simulink model "Rider_Controls_OutHardware"  (R2014b)
settings: configuration reference "Embedded_Configuration" (kept outside this file)
PostLoadFcn:
  | load('Embedded_Config.mat')
model workspace: external: MAT-File Embedded_Config.mat (data not in the file)
libraries: canmsglib x2, c280xlib x2
settings Model: Creator=The MathWorks Inc.  LastModifiedBy=Sean

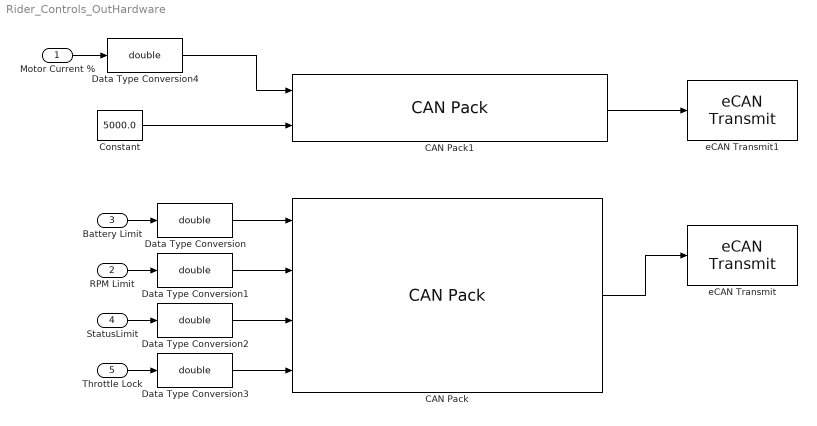
== system Rider_Controls_OutHardware ==
  Motor Current % : Inport  OutDataTypeStr=single
  RPM Limit : Inport  Port=2  OutDataTypeStr=uint16
  Battery Limit : Inport  Port=3  OutDataTypeStr=uint16
  StatusLimit : Inport  Port=4  OutDataTypeStr=uint16
  Throttle Lock : Inport  Port=5  OutDataTypeStr=uint16
  CAN Pack : canmsglib/CAN Pack  CANdbFile=C:\Users\Sean\Desktop\Buckeye Current\Databases\RW3.dbc  MsgList=DriveControlsLimits  MsgName=DriveControlsLimits  MsgIDType=Standard (11-bit identifier)  MsgIdentifier=483  MsgLength=8  SignalInfo=BatteryLimit$1$1$1$2$1$0$1$0$0$1$#RPMLimit$2$1$1$2$1$0$1$0$0$1$#StatusLimit$3$1$1$2$1$0$1$0$-Inf$Inf$#ThrottleLock$0$1$1$2$1$0$1$0$-Inf$Inf$#  NSignals=4  StartBits=str2num('[int32(1);int32(2);int32(3);int32(0)]')  SignalSizes=str2num('[int32(1);int32(1);int32(1);int32(1)]')  ByteOrders=str2num('[int32(1);int32(1);int32(1);int32(1)]')  DataTypes=str2num('[int32(2);int32(2);int32(2);int32(2)]')  MultiplexTypes=str2num('[int32(1);int32(1);int32(1);int32(1)]')  MultiplexValues=str2num('[double(0);double(0);double(0);double(0)]')  Factors=str2num('[double(1);double(1);double(1);double(1)]')  Offsets=str2num('[double(0);double(0);double(0);double(0)]')  Minimums=str2num('[double(0);double(0);double(-Inf);double(-Inf)]')  Maximums=str2num('[double(1);double(1);double(Inf);double(Inf)]')  Remote=off
      settings: DataFormat=CANdb specified signals
  CAN Pack1 : canmsglib/CAN Pack  CANdbFile=C:\Users\Sean\Desktop\Buckeye Current\Databases\RW3.dbc  MsgList=MotorDriveCommand  MsgName=MotorDriveCommand  MsgIDType=Standard (11-bit identifier)  MsgIdentifier=480  MsgLength=8  SignalInfo=MotorCurrentSetpoint$32$32$1$3$1$0$1$0$0$1$#MotorRPMSetpoint$0$32$1$3$1$0$1$0$0$4000$#  NSignals=2  StartBits=str2num('[int32(32);int32(0)]')  SignalSizes=str2num('[int32(32);int32(32)]')  ByteOrders=str2num('[int32(1);int32(1)]')  DataTypes=str2num('[int32(3);int32(3)]')  MultiplexTypes=str2num('[int32(1);int32(1)]')  MultiplexValues=str2num('[double(0);double(0)]')  Factors=str2num('[double(1);double(1)]')  Offsets=str2num('[double(0);double(0)]')  Minimums=str2num('[double(0);double(0)]')  Maximums=str2num('[double(1);double(4000)]')  Remote=off
      settings: DataFormat=CANdb specified signals
  Constant : Constant  Value=5000.0  OutDataTypeStr=Inherit: Inherit via back propagation  SampleTime=0.01
  Data Type Conversion{,1..4} (5 alike) : DataTypeConversion  OutDataTypeStr=double
  eCAN Transmit : c280xlib/eCAN Transmit  chipFamily=C280x  useModule=eCAN_A  mailboxNo=31  messageID=483  messageType=Standard (11-bit identifier)  enableBlockingMode=off  postInterrupt=off  interruptLine=0
  eCAN Transmit1 : c280xlib/eCAN Transmit  chipFamily=C280x  useModule=eCAN_A  mailboxNo=30  messageID=480  messageType=Standard (11-bit identifier)  enableBlockingMode=off  postInterrupt=off  interruptLine=0
  wires:
  Battery Limit/1 -> Data Type Conversion/1
  RPM Limit/1 -> Data Type Conversion1/1
  Motor Current %/1 -> Data Type Conversion4/1
  Constant/1 -> CAN Pack1/2
  CAN Pack/1 -> eCAN Transmit/1
  Throttle Lock/1 -> Data Type Conversion3/1
  StatusLimit/1 -> Data Type Conversion2/1
  Data Type Conversion/1 -> CAN Pack/1
  Data Type Conversion1/1 -> CAN Pack/2
  Data Type Conversion2/1 -> CAN Pack/3
  Data Type Conversion3/1 -> CAN Pack/4
  Data Type Conversion4/1 -> CAN Pack1/1
  CAN Pack1/1 -> eCAN Transmit1/1
